simulink model "qconv"  (Simulink 8.6)
settings: Solver=FixedStepDiscrete  StartTime=0.0  StopTime=1  FixedStep=dt  RelTol=1e-3
InitFcn:
  | param
values from neighbouring files (symbols this model uses):
  ampl = 5    [param.m]
  dt = 0.00005    (= 5e-05)    [param.m]
  freq = 5000    [param.m]
  phi0 = pi/4    (= 0.785398163397)    [param.m]
  T = 0.15    [param.m]
undefined symbols (not defined in the file or in its folder): DiscIntNeverNeededParam
libraries: qconvolution x6, commchan3 x1
settings Model: Creator=m.rodkin  LastModifiedBy=mishuk
settings OptimizationCC: DefaultParameterBehavior=Inlined  InlineInvariantSignals=on
settings DebuggingCC: FcnCallInpInsideContextMsg=EnableAllAsWarning

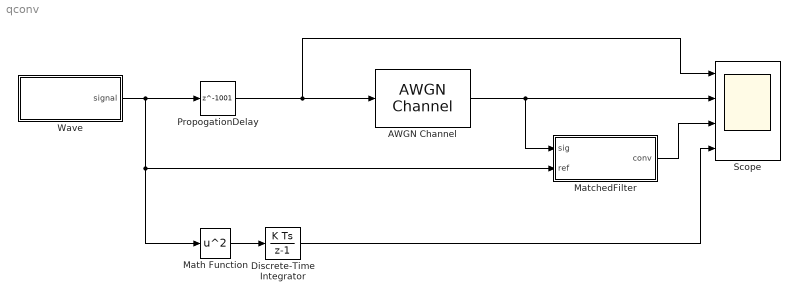
== system qconv ==
  AWGN Channel : commchan3/AWGN Channel  InputProcessing=Columns as channels (frame based)  seed=67  noiseMode=Variance from mask  EbNodB=10  EsNodB=10  SNRdB=0  bitsPerSym=1  Ps=0.01  Tsym=1  variance=noiseVariance
  Discrete-Time Integrator : DiscreteIntegrator  SampleTime=dt  ICPrevOutput=DiscIntNeverNeededParam  ICPrevScaledInput=DiscIntNeverNeededParam
  MatchedFilter : Subsystem
  Math Function : Math  Operator=square  SampleTime=dt  SaturateOnIntegerOverflow=on
  PropogationDelay : Delay  DelayLength=1001
  Scope : Scope  NumInputPorts=4
  Wave : Subsystem
  wires:
  AWGN Channel/1 -> Scope/2, MatchedFilter/1(sig)
  MatchedFilter/1(conv) -> Scope/3
  Wave/1(signal) -> PropogationDelay/1, Math Function/1, MatchedFilter/2(ref)
  PropogationDelay/1 -> AWGN Channel/1, Scope/1
  Math Function/1 -> Discrete-Time Integrator/1
  Discrete-Time Integrator/1 -> Scope/4

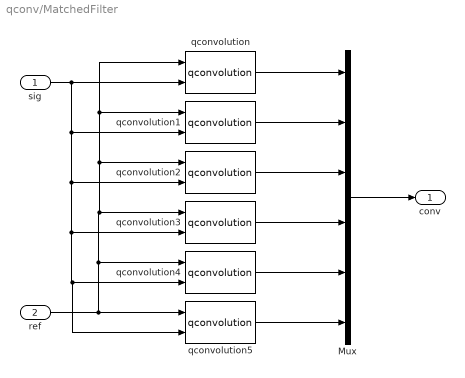
== system qconv/MatchedFilter ==
  sig : Inport
  ref : Inport  Port=2
  Mux : Mux  Inputs=6
  qconvolution : qconvolution/qconvolution  delay=1000
  qconvolution1 : qconvolution/qconvolution  delay=2500
  qconvolution2 : qconvolution/qconvolution  delay=4000
  qconvolution3 : qconvolution/qconvolution  delay=5500
  qconvolution4 : qconvolution/qconvolution  delay=7000
  qconvolution5 : qconvolution/qconvolution  delay=8500
  conv : Outport
  wires:
  Mux/1 -> conv/1
  sig/1 -> qconvolution/2, qconvolution1/2, qconvolution2/2, qconvolution3/2, qconvolution5/2, qconvolution4/2
  qconvolution5/1 -> Mux/6
  qconvolution4/1 -> Mux/5
  qconvolution/1 -> Mux/1
  qconvolution1/1 -> Mux/2
  qconvolution2/1 -> Mux/3
  qconvolution3/1 -> Mux/4
  ref/1 -> qconvolution5/1, qconvolution4/1, qconvolution3/1, qconvolution2/1, qconvolution/1, qconvolution1/1

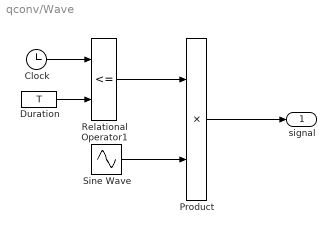
== system qconv/Wave ==
  Clock : Clock
  Duration : Constant  Value=T
  Product : Product  RndMeth=Zero
  Relational Operator1 : RelationalOperator  Operator=<=  OutDataTypeStr=boolean
  Sine Wave : Sin  Amplitude=ampl  Frequency=2*pi*freq  Phase=phi0  SampleTime=dt
  signal : Outport
  wires:
  Duration/1 -> Relational Operator1/2
  Product/1 -> signal/1
  Clock/1 -> Relational Operator1/1
  Sine Wave/1 -> Product/2
  Relational Operator1/1 -> Product/1
